simulink model "eVTOL_System"  (R2024b)
settings: Solver=FixedStepAuto  StartTime=0.0  StopTime=inf  RelTol=1e-3
undefined symbols (not defined in the file): airspeed, Battery, BCE12, BCE_Set_init, BMS_Controller_State, C, Cell10_P, Cell11_P, Cell12_P, Cell13_P, Cell14_P, Cell15_P, Cell16_P, Cell17_P, Cell18_P, Cell19_P, Cell1_N, Cell1_P, Cell20_P, Cell21_P, Cell22_P, Cell23_P, Cell24_P, Cell2_P, Cell3_P, Cell4_P, Cell5_P, Cell6_P, Cell7_P, Cell8_P, Cell9_P, Charging_State, CityMission, control, controlParams, ControlSampleTime, CriticalTiltAngle, currentFactor, CV_Gain, ddx, ddy, ddz, Device_01, Device_02, DiscIntNeverNeededParam, dx, dy, dz, Earth, env, F, F28379D_ADC_MaxCount, F28379D_ADC_Vmax, FixedWingMission, flightState, Foc_Ki_IxTcpu, Foc_Ki_S, Foc_Kp_I, Foc_Kp_S, fractalcoef ... (+68)
libraries: fl_lib x1115, nesl_utility x617, slrealtimeethercatlib x217, simulink x130, canmsglib x101, speedgoatlib_IO611_obsolete x91, slpidlib x49, mcbcontrolslib x44, slrealtimeutilitieslib x35, speedgoatlib_hdlCoder_IO3xx x31, dspstat3 x24, mcbpositiondecoderlib x12
(part 2 of 31)

== system eVTOL_System/Motor Drive/Controller3 ==
  Iab : Inport
  QAE_MIL_fbk : Inport  Port=2
  EnablePWM : Inport  Port=3
  Closed_Loop_FOC : Inport  Port=4
  Speed_CMD_RPM : Inport  Port=5
  Controller_Parameters : Inport  Port=6
  Controller_MIL : Subsystem  VariantControl=(default)
  Controller_fbk : Outport
  Simu_config : Outport  Port=2

== system eVTOL_System/Motor Drive/Controller_fbk_signals ==
  Controller_fbk : Inport
  Data Type Conversion : DataTypeConversion  OutDataTypeStr=boolean  SaturateOnIntegerOverflow=off  RndMeth=Floor
  Demux : Demux
  Terminator{,1..3} (4 alike) : Terminator
  wires:
  Demux/1 -> Terminator1/1  "Speed_fbk"
  Controller_fbk/1 -> Demux/1
  Demux/2 -> Terminator3/1  "Encoder_Pos_fbk"
  Demux/4 -> Data Type Conversion/1  "Spd_Pot_fdk"
  Demux/3 -> Terminator2/1  "Speed_Cmd_fbk"
  Data Type Conversion/1 -> Terminator/1  "Spd_pot_enable"

== system eVTOL_System/Motor Drive/Controller_fbk_signals1 ==
  Controller_fbk : Inport
  Data Type Conversion : DataTypeConversion  OutDataTypeStr=boolean  SaturateOnIntegerOverflow=off  RndMeth=Floor
  Demux : Demux
  Terminator{,1..3} (4 alike) : Terminator
  wires:
  Demux/1 -> Terminator1/1  "Speed_fbk"
  Controller_fbk/1 -> Demux/1
  Demux/2 -> Terminator3/1  "Encoder_Pos_fbk"
  Demux/4 -> Data Type Conversion/1  "Spd_Pot_fdk"
  Demux/3 -> Terminator2/1  "Speed_Cmd_fbk"
  Data Type Conversion/1 -> Terminator/1  "Spd_pot_enable"

== system eVTOL_System/Motor Drive/Controller_fbk_signals2 ==
  Controller_fbk : Inport
  Data Type Conversion : DataTypeConversion  OutDataTypeStr=boolean  SaturateOnIntegerOverflow=off  RndMeth=Floor
  Demux : Demux
  Terminator{,1..3} (4 alike) : Terminator
  wires:
  Demux/1 -> Terminator1/1  "Speed_fbk"
  Controller_fbk/1 -> Demux/1
  Demux/2 -> Terminator3/1  "Encoder_Pos_fbk"
  Demux/4 -> Data Type Conversion/1  "Spd_Pot_fdk"
  Demux/3 -> Terminator2/1  "Speed_Cmd_fbk"
  Data Type Conversion/1 -> Terminator/1  "Spd_pot_enable"

== system eVTOL_System/Motor Drive/Controller_fbk_signals3 ==
  Controller_fbk : Inport
  Data Type Conversion : DataTypeConversion  OutDataTypeStr=boolean  SaturateOnIntegerOverflow=off  RndMeth=Floor
  Demux : Demux
  Terminator{,1..3} (4 alike) : Terminator
  wires:
  Demux/1 -> Terminator1/1  "Speed_fbk"
  Controller_fbk/1 -> Demux/1
  Demux/2 -> Terminator3/1  "Encoder_Pos_fbk"
  Demux/4 -> Data Type Conversion/1  "Spd_Pot_fdk"
  Demux/3 -> Terminator2/1  "Speed_Cmd_fbk"
  Data Type Conversion/1 -> Terminator/1  "Spd_pot_enable"

== system eVTOL_System/Motor Drive/Fault Trigering ==
  AND : Logic  Inputs=3  IconShape=distinctive  AllPortsSameDT=off  OutDataTypeStr=boolean
  Bit to Integer Converter : simulink/Logic and Bit Operations/Bit to Integer Converter  nbits=32  bitOrder=LSB first  signedOutputValues=Unsigned  outDtype=uint32  outDtypeSigned=Inherit via internal rule
  Close_An : Constant  Value=0  OutDataTypeStr=boolean  SampleTime=Ts_UI
  Close_Ap : Constant  Value=0  OutDataTypeStr=boolean  SampleTime=Ts_UI
  Close_Bn : Constant  Value=0  OutDataTypeStr=boolean  SampleTime=Ts_UI
  Close_Bp : Constant  Value=0  OutDataTypeStr=boolean  SampleTime=Ts_UI
  Close_Cn : Constant  Value=0  OutDataTypeStr=boolean  SampleTime=Ts_UI
  Close_Cp : Constant  Value=0  OutDataTypeStr=boolean  SampleTime=Ts_UI
  Constant1 : Constant  Value=0  OutDataTypeStr=uint32
  Constant{14..15,20..25,32..36} (13 alike) : Constant  Value=0  OutDataTypeStr=boolean  SampleTime=Ts_UI
  Constant2 : Constant  OutDataTypeStr=boolean  SampleTime=Ts_UI
  Enable_Fault_UI : Constant  OutDataTypeStr=boolean  SampleTime=Ts_UI
  OR : Logic  Operator=OR  Inputs=18  IconShape=distinctive  AllPortsSameDT=off  OutDataTypeStr=boolean
  Open_An : Constant  Value=0  OutDataTypeStr=boolean  SampleTime=Ts_UI
  Open_Ap : Constant  Value=0  OutDataTypeStr=boolean  SampleTime=Ts_UI
  Open_Bn : Constant  Value=0  OutDataTypeStr=boolean  SampleTime=Ts_UI
  Open_Bp : Constant  Value=0  OutDataTypeStr=boolean  SampleTime=Ts_UI
  Open_Cn : Constant  Value=0  OutDataTypeStr=boolean  SampleTime=Ts_UI
  Open_Cp : Constant  Value=0  OutDataTypeStr=boolean  SampleTime=Ts_UI
  Short_A : Constant  Value=0  OutDataTypeStr=boolean  SampleTime=Ts_UI
  Short_AB : Constant  Value=0  OutDataTypeStr=boolean  SampleTime=Ts_UI
  Short_B : Constant  Value=0  OutDataTypeStr=boolean  SampleTime=Ts_UI
  Short_BC : Constant  Value=0  OutDataTypeStr=boolean  SampleTime=Ts_UI
  Short_C : Constant  Value=0  OutDataTypeStr=boolean  SampleTime=Ts_UI
  Short_CA : Constant  Value=0  OutDataTypeStr=boolean  SampleTime=Ts_UI
  Switch : Switch  Criteria=u2 > Threshold  SaturateOnIntegerOverflow=off  InputSameDT=off
  Terminator : Terminator
  Vector Concatenate : Concatenate  NumInputs=32
  Faults : Outport
  wires:
  Open_Cn/1 -> OR/12, Vector Concatenate/12
  Open_Cp/1 -> OR/9, Vector Concatenate/9
  Short_A/1 -> OR/1, Vector Concatenate/1
  Open_Bp/1 -> OR/8, Vector Concatenate/8
  Short_B/1 -> Vector Concatenate/2, OR/2
  Short_C/1 -> Vector Concatenate/3, OR/3
  Short_AB/1 -> Vector Concatenate/4, OR/4
  Short_BC/1 -> Vector Concatenate/5, OR/5
  Short_CA/1 -> OR/6, Vector Concatenate/6
  Constant36/1 -> Vector Concatenate/31
  Open_Bn/1 -> OR/11, Vector Concatenate/11
  Open_An/1 -> OR/10, Vector Concatenate/10
  Open_Ap/1 -> OR/7, Vector Concatenate/7
  Close_An/1 -> OR/16, Vector Concatenate/16
  Close_Ap/1 -> OR/13, Vector Concatenate/13
  Close_Cn/1 -> OR/18, Vector Concatenate/18
  Close_Bn/1 -> OR/17, Vector Concatenate/17
  Close_Cp/1 -> OR/15, Vector Concatenate/15
  Close_Bp/1 -> OR/14, Vector Concatenate/14
  Constant15/1 -> Vector Concatenate/24
  Constant14/1 -> Vector Concatenate/23
  Constant21/1 -> Vector Concatenate/20
  Constant20/1 -> Vector Concatenate/19
  Constant25/1 -> Vector Concatenate/26
  Constant24/1 -> Vector Concatenate/25
  Constant23/1 -> Vector Concatenate/22
  Constant22/1 -> Vector Concatenate/21
  Constant35/1 -> Vector Concatenate/30
  Constant34/1 -> Vector Concatenate/29
  Constant33/1 -> Vector Concatenate/28
  Constant32/1 -> Vector Concatenate/27
  Enable_Fault_UI/1 -> AND/3, Switch/2
  Vector Concatenate/1 -> Bit to Integer Converter/1
  Switch/1 -> Faults/1
  Bit to Integer Converter/1 -> Switch/1
  Constant1/1 -> Switch/3
  OR/1 -> AND/1
  AND/1 -> Terminator/1  "Fault_Present"
  Constant2/1 -> AND/2, Vector Concatenate/32

== system eVTOL_System/Motor Drive/Fault Trigering1 ==
  AND : Logic  Inputs=3  IconShape=distinctive  AllPortsSameDT=off  OutDataTypeStr=boolean
  Bit to Integer Converter : simulink/Logic and Bit Operations/Bit to Integer Converter  nbits=32  bitOrder=LSB first  signedOutputValues=Unsigned  outDtype=uint32  outDtypeSigned=Inherit via internal rule
  Close_An : Constant  Value=0  OutDataTypeStr=boolean  SampleTime=Ts_UI
  Close_Ap : Constant  Value=0  OutDataTypeStr=boolean  SampleTime=Ts_UI
  Close_Bn : Constant  Value=0  OutDataTypeStr=boolean  SampleTime=Ts_UI
  Close_Bp : Constant  Value=0  OutDataTypeStr=boolean  SampleTime=Ts_UI
  Close_Cn : Constant  Value=0  OutDataTypeStr=boolean  SampleTime=Ts_UI
  Close_Cp : Constant  Value=0  OutDataTypeStr=boolean  SampleTime=Ts_UI
  Constant1 : Constant  Value=0  OutDataTypeStr=uint32
  Constant{14..15,20..25,32..36} (13 alike) : Constant  Value=0  OutDataTypeStr=boolean  SampleTime=Ts_UI
  Constant2 : Constant  OutDataTypeStr=boolean  SampleTime=Ts_UI
  Enable_Fault_UI : Constant  OutDataTypeStr=boolean  SampleTime=Ts_UI
  OR : Logic  Operator=OR  Inputs=18  IconShape=distinctive  AllPortsSameDT=off  OutDataTypeStr=boolean
  Open_An : Constant  Value=0  OutDataTypeStr=boolean  SampleTime=Ts_UI
  Open_Ap : Constant  Value=0  OutDataTypeStr=boolean  SampleTime=Ts_UI
  Open_Bn : Constant  Value=0  OutDataTypeStr=boolean  SampleTime=Ts_UI
  Open_Bp : Constant  Value=0  OutDataTypeStr=boolean  SampleTime=Ts_UI
  Open_Cn : Constant  Value=0  OutDataTypeStr=boolean  SampleTime=Ts_UI
  Open_Cp : Constant  Value=0  OutDataTypeStr=boolean  SampleTime=Ts_UI
  Short_A : Constant  Value=0  OutDataTypeStr=boolean  SampleTime=Ts_UI
  Short_AB : Constant  Value=0  OutDataTypeStr=boolean  SampleTime=Ts_UI
  Short_B : Constant  Value=0  OutDataTypeStr=boolean  SampleTime=Ts_UI
  Short_BC : Constant  Value=0  OutDataTypeStr=boolean  SampleTime=Ts_UI
  Short_C : Constant  Value=0  OutDataTypeStr=boolean  SampleTime=Ts_UI
  Short_CA : Constant  Value=0  OutDataTypeStr=boolean  SampleTime=Ts_UI
  Switch : Switch  Criteria=u2 > Threshold  SaturateOnIntegerOverflow=off  InputSameDT=off
  Terminator : Terminator
  Vector Concatenate : Concatenate  NumInputs=32
  Faults : Outport
  wires:
  Open_Cn/1 -> OR/12, Vector Concatenate/12
  Open_Cp/1 -> OR/9, Vector Concatenate/9
  Short_A/1 -> OR/1, Vector Concatenate/1
  Open_Bp/1 -> OR/8, Vector Concatenate/8
  Short_B/1 -> Vector Concatenate/2, OR/2
  Short_C/1 -> Vector Concatenate/3, OR/3
  Short_AB/1 -> Vector Concatenate/4, OR/4
  Short_BC/1 -> Vector Concatenate/5, OR/5
  Short_CA/1 -> OR/6, Vector Concatenate/6
  Constant36/1 -> Vector Concatenate/31
  Open_Bn/1 -> OR/11, Vector Concatenate/11
  Open_An/1 -> OR/10, Vector Concatenate/10
  Open_Ap/1 -> OR/7, Vector Concatenate/7
  Close_An/1 -> OR/16, Vector Concatenate/16
  Close_Ap/1 -> OR/13, Vector Concatenate/13
  Close_Cn/1 -> OR/18, Vector Concatenate/18
  Close_Bn/1 -> OR/17, Vector Concatenate/17
  Close_Cp/1 -> OR/15, Vector Concatenate/15
  Close_Bp/1 -> OR/14, Vector Concatenate/14
  Constant15/1 -> Vector Concatenate/24
  Constant14/1 -> Vector Concatenate/23
  Constant21/1 -> Vector Concatenate/20
  Constant20/1 -> Vector Concatenate/19
  Constant25/1 -> Vector Concatenate/26
  Constant24/1 -> Vector Concatenate/25
  Constant23/1 -> Vector Concatenate/22
  Constant22/1 -> Vector Concatenate/21
  Constant35/1 -> Vector Concatenate/30
  Constant34/1 -> Vector Concatenate/29
  Constant33/1 -> Vector Concatenate/28
  Constant32/1 -> Vector Concatenate/27
  Enable_Fault_UI/1 -> AND/3, Switch/2
  Vector Concatenate/1 -> Bit to Integer Converter/1
  Switch/1 -> Faults/1
  Bit to Integer Converter/1 -> Switch/1
  Constant1/1 -> Switch/3
  OR/1 -> AND/1
  AND/1 -> Terminator/1  "Fault_Present"
  Constant2/1 -> AND/2, Vector Concatenate/32

== system eVTOL_System/Motor Drive/Fault Trigering2 ==
  AND : Logic  Inputs=3  IconShape=distinctive  AllPortsSameDT=off  OutDataTypeStr=boolean
  Bit to Integer Converter : simulink/Logic and Bit Operations/Bit to Integer Converter  nbits=32  bitOrder=LSB first  signedOutputValues=Unsigned  outDtype=uint32  outDtypeSigned=Inherit via internal rule
  Close_An : Constant  Value=0  OutDataTypeStr=boolean  SampleTime=Ts_UI
  Close_Ap : Constant  Value=0  OutDataTypeStr=boolean  SampleTime=Ts_UI
  Close_Bn : Constant  Value=0  OutDataTypeStr=boolean  SampleTime=Ts_UI
  Close_Bp : Constant  Value=0  OutDataTypeStr=boolean  SampleTime=Ts_UI
  Close_Cn : Constant  Value=0  OutDataTypeStr=boolean  SampleTime=Ts_UI
  Close_Cp : Constant  Value=0  OutDataTypeStr=boolean  SampleTime=Ts_UI
  Constant1 : Constant  Value=0  OutDataTypeStr=uint32
  Constant{14..15,20..25,32..36} (13 alike) : Constant  Value=0  OutDataTypeStr=boolean  SampleTime=Ts_UI
  Constant2 : Constant  OutDataTypeStr=boolean  SampleTime=Ts_UI
  Enable_Fault_UI : Constant  OutDataTypeStr=boolean  SampleTime=Ts_UI
  OR : Logic  Operator=OR  Inputs=18  IconShape=distinctive  AllPortsSameDT=off  OutDataTypeStr=boolean
  Open_An : Constant  Value=0  OutDataTypeStr=boolean  SampleTime=Ts_UI
  Open_Ap : Constant  Value=0  OutDataTypeStr=boolean  SampleTime=Ts_UI
  Open_Bn : Constant  Value=0  OutDataTypeStr=boolean  SampleTime=Ts_UI
  Open_Bp : Constant  Value=0  OutDataTypeStr=boolean  SampleTime=Ts_UI
  Open_Cn : Constant  Value=0  OutDataTypeStr=boolean  SampleTime=Ts_UI
  Open_Cp : Constant  Value=0  OutDataTypeStr=boolean  SampleTime=Ts_UI
  Short_A : Constant  Value=0  OutDataTypeStr=boolean  SampleTime=Ts_UI
  Short_AB : Constant  Value=0  OutDataTypeStr=boolean  SampleTime=Ts_UI
  Short_B : Constant  Value=0  OutDataTypeStr=boolean  SampleTime=Ts_UI
  Short_BC : Constant  Value=0  OutDataTypeStr=boolean  SampleTime=Ts_UI
  Short_C : Constant  Value=0  OutDataTypeStr=boolean  SampleTime=Ts_UI
  Short_CA : Constant  Value=0  OutDataTypeStr=boolean  SampleTime=Ts_UI
  Switch : Switch  Criteria=u2 > Threshold  SaturateOnIntegerOverflow=off  InputSameDT=off
  Terminator : Terminator
  Vector Concatenate : Concatenate  NumInputs=32
  Faults : Outport
  wires:
  Open_Cn/1 -> OR/12, Vector Concatenate/12
  Open_Cp/1 -> OR/9, Vector Concatenate/9
  Short_A/1 -> OR/1, Vector Concatenate/1
  Open_Bp/1 -> OR/8, Vector Concatenate/8
  Short_B/1 -> Vector Concatenate/2, OR/2
  Short_C/1 -> Vector Concatenate/3, OR/3
  Short_AB/1 -> Vector Concatenate/4, OR/4
  Short_BC/1 -> Vector Concatenate/5, OR/5
  Short_CA/1 -> OR/6, Vector Concatenate/6
  Constant36/1 -> Vector Concatenate/31
  Open_Bn/1 -> OR/11, Vector Concatenate/11
  Open_An/1 -> OR/10, Vector Concatenate/10
  Open_Ap/1 -> OR/7, Vector Concatenate/7
  Close_An/1 -> OR/16, Vector Concatenate/16
  Close_Ap/1 -> OR/13, Vector Concatenate/13
  Close_Cn/1 -> OR/18, Vector Concatenate/18
  Close_Bn/1 -> OR/17, Vector Concatenate/17
  Close_Cp/1 -> OR/15, Vector Concatenate/15
  Close_Bp/1 -> OR/14, Vector Concatenate/14
  Constant15/1 -> Vector Concatenate/24
  Constant14/1 -> Vector Concatenate/23
  Constant21/1 -> Vector Concatenate/20
  Constant20/1 -> Vector Concatenate/19
  Constant25/1 -> Vector Concatenate/26
  Constant24/1 -> Vector Concatenate/25
  Constant23/1 -> Vector Concatenate/22
  Constant22/1 -> Vector Concatenate/21
  Constant35/1 -> Vector Concatenate/30
  Constant34/1 -> Vector Concatenate/29
  Constant33/1 -> Vector Concatenate/28
  Constant32/1 -> Vector Concatenate/27
  Enable_Fault_UI/1 -> AND/3, Switch/2
  Vector Concatenate/1 -> Bit to Integer Converter/1
  Switch/1 -> Faults/1
  Bit to Integer Converter/1 -> Switch/1
  Constant1/1 -> Switch/3
  OR/1 -> AND/1
  AND/1 -> Terminator/1  "Fault_Present"
  Constant2/1 -> AND/2, Vector Concatenate/32

== system eVTOL_System/Motor Drive/Fault Trigering3 ==
  AND : Logic  Inputs=3  IconShape=distinctive  AllPortsSameDT=off  OutDataTypeStr=boolean
  Bit to Integer Converter : simulink/Logic and Bit Operations/Bit to Integer Converter  nbits=32  bitOrder=LSB first  signedOutputValues=Unsigned  outDtype=uint32  outDtypeSigned=Inherit via internal rule
  Close_An : Constant  Value=0  OutDataTypeStr=boolean  SampleTime=Ts_UI
  Close_Ap : Constant  Value=0  OutDataTypeStr=boolean  SampleTime=Ts_UI
  Close_Bn : Constant  Value=0  OutDataTypeStr=boolean  SampleTime=Ts_UI
  Close_Bp : Constant  Value=0  OutDataTypeStr=boolean  SampleTime=Ts_UI
  Close_Cn : Constant  Value=0  OutDataTypeStr=boolean  SampleTime=Ts_UI
  Close_Cp : Constant  Value=0  OutDataTypeStr=boolean  SampleTime=Ts_UI
  Constant1 : Constant  Value=0  OutDataTypeStr=uint32
  Constant{14..15,20..25,32..36} (13 alike) : Constant  Value=0  OutDataTypeStr=boolean  SampleTime=Ts_UI
  Constant2 : Constant  OutDataTypeStr=boolean  SampleTime=Ts_UI
  Enable_Fault_UI : Constant  OutDataTypeStr=boolean  SampleTime=Ts_UI
  OR : Logic  Operator=OR  Inputs=18  IconShape=distinctive  AllPortsSameDT=off  OutDataTypeStr=boolean
  Open_An : Constant  Value=0  OutDataTypeStr=boolean  SampleTime=Ts_UI
  Open_Ap : Constant  Value=0  OutDataTypeStr=boolean  SampleTime=Ts_UI
  Open_Bn : Constant  Value=0  OutDataTypeStr=boolean  SampleTime=Ts_UI
  Open_Bp : Constant  Value=0  OutDataTypeStr=boolean  SampleTime=Ts_UI
  Open_Cn : Constant  Value=0  OutDataTypeStr=boolean  SampleTime=Ts_UI
  Open_Cp : Constant  Value=0  OutDataTypeStr=boolean  SampleTime=Ts_UI
  Short_A : Constant  Value=0  OutDataTypeStr=boolean  SampleTime=Ts_UI
  Short_AB : Constant  Value=0  OutDataTypeStr=boolean  SampleTime=Ts_UI
  Short_B : Constant  Value=0  OutDataTypeStr=boolean  SampleTime=Ts_UI
  Short_BC : Constant  Value=0  OutDataTypeStr=boolean  SampleTime=Ts_UI
  Short_C : Constant  Value=0  OutDataTypeStr=boolean  SampleTime=Ts_UI
  Short_CA : Constant  Value=0  OutDataTypeStr=boolean  SampleTime=Ts_UI
  Switch : Switch  Criteria=u2 > Threshold  SaturateOnIntegerOverflow=off  InputSameDT=off
  Terminator : Terminator
  Vector Concatenate : Concatenate  NumInputs=32
  Faults : Outport
  wires:
  Open_Cn/1 -> OR/12, Vector Concatenate/12
  Open_Cp/1 -> OR/9, Vector Concatenate/9
  Short_A/1 -> OR/1, Vector Concatenate/1
  Open_Bp/1 -> OR/8, Vector Concatenate/8
  Short_B/1 -> Vector Concatenate/2, OR/2
  Short_C/1 -> Vector Concatenate/3, OR/3
  Short_AB/1 -> Vector Concatenate/4, OR/4
  Short_BC/1 -> Vector Concatenate/5, OR/5
  Short_CA/1 -> OR/6, Vector Concatenate/6
  Constant36/1 -> Vector Concatenate/31
  Open_Bn/1 -> OR/11, Vector Concatenate/11
  Open_An/1 -> OR/10, Vector Concatenate/10
  Open_Ap/1 -> OR/7, Vector Concatenate/7
  Close_An/1 -> OR/16, Vector Concatenate/16
  Close_Ap/1 -> OR/13, Vector Concatenate/13
  Close_Cn/1 -> OR/18, Vector Concatenate/18
  Close_Bn/1 -> OR/17, Vector Concatenate/17
  Close_Cp/1 -> OR/15, Vector Concatenate/15
  Close_Bp/1 -> OR/14, Vector Concatenate/14
  Constant15/1 -> Vector Concatenate/24
  Constant14/1 -> Vector Concatenate/23
  Constant21/1 -> Vector Concatenate/20
  Constant20/1 -> Vector Concatenate/19
  Constant25/1 -> Vector Concatenate/26
  Constant24/1 -> Vector Concatenate/25
  Constant23/1 -> Vector Concatenate/22
  Constant22/1 -> Vector Concatenate/21
  Constant35/1 -> Vector Concatenate/30
  Constant34/1 -> Vector Concatenate/29
  Constant33/1 -> Vector Concatenate/28
  Constant32/1 -> Vector Concatenate/27
  Enable_Fault_UI/1 -> AND/3, Switch/2
  Vector Concatenate/1 -> Bit to Integer Converter/1
  Switch/1 -> Faults/1
  Bit to Integer Converter/1 -> Switch/1
  Constant1/1 -> Switch/3
  OR/1 -> AND/1
  AND/1 -> Terminator/1  "Fault_Present"
  Constant2/1 -> AND/2, Vector Concatenate/32

== system eVTOL_System/Motor Drive/Motor Model Feedback ==
  Ia : Inport
  Ib : Inport  Port=2
  Ic : Inport  Port=3
  Motor_SPD_rads : Inport  Port=4
  Rate Transition{,1..3} (4 alike) : RateTransition  OutPortSampleTime=Ts_UI_fast
  Terminator{,1..3} (4 alike) : Terminator
  radsTOrpm : Gain  Gain=60/(2*pi)
  wires:
  Rate Transition1/1 -> Terminator/1  "Ia"
  Rate Transition3/1 -> Terminator2/1  "Ic"
  Rate Transition2/1 -> Terminator1/1  "Ib"
  Ib/1 -> Rate Transition2/1
  Ia/1 -> Rate Transition1/1
  Ic/1 -> Rate Transition3/1
  Motor_SPD_rads/1 -> Rate Transition/1
  radsTOrpm/1 -> Terminator3/1  "Motor Speed RPM"
  Rate Transition/1 -> radsTOrpm/1

== system eVTOL_System/Motor Drive/Motor Model Feedback1 ==
  Ia : Inport
  Ib : Inport  Port=2
  Ic : Inport  Port=3
  Motor_SPD_rads : Inport  Port=4
  Rate Transition{,1..3} (4 alike) : RateTransition  OutPortSampleTime=Ts_UI_fast
  Terminator{,1..3} (4 alike) : Terminator
  radsTOrpm : Gain  Gain=60/(2*pi)
  wires:
  Rate Transition1/1 -> Terminator/1  "Ia"
  Rate Transition3/1 -> Terminator2/1  "Ic"
  Rate Transition2/1 -> Terminator1/1  "Ib"
  Ib/1 -> Rate Transition2/1
  Ia/1 -> Rate Transition1/1
  Ic/1 -> Rate Transition3/1
  Motor_SPD_rads/1 -> Rate Transition/1
  radsTOrpm/1 -> Terminator3/1  "Motor Speed RPM"
  Rate Transition/1 -> radsTOrpm/1

== system eVTOL_System/Motor Drive/Motor Model Feedback2 ==
  Ia : Inport
  Ib : Inport  Port=2
  Ic : Inport  Port=3
  Motor_SPD_rads : Inport  Port=4
  Rate Transition{,1..3} (4 alike) : RateTransition  OutPortSampleTime=Ts_UI_fast
  Terminator{,1..3} (4 alike) : Terminator
  radsTOrpm : Gain  Gain=60/(2*pi)
  wires:
  Rate Transition1/1 -> Terminator/1  "Ia"
  Rate Transition3/1 -> Terminator2/1  "Ic"
  Rate Transition2/1 -> Terminator1/1  "Ib"
  Ib/1 -> Rate Transition2/1
  Ia/1 -> Rate Transition1/1
  Ic/1 -> Rate Transition3/1
  Motor_SPD_rads/1 -> Rate Transition/1
  radsTOrpm/1 -> Terminator3/1  "Motor Speed RPM"
  Rate Transition/1 -> radsTOrpm/1

== system eVTOL_System/Motor Drive/Motor Model Feedback3 ==
  Ia : Inport
  Ib : Inport  Port=2
  Ic : Inport  Port=3
  Motor_SPD_rads : Inport  Port=4
  Rate Transition{,1..3} (4 alike) : RateTransition  OutPortSampleTime=Ts_UI_fast
  Terminator{,1..3} (4 alike) : Terminator
  radsTOrpm : Gain  Gain=60/(2*pi)
  wires:
  Rate Transition1/1 -> Terminator/1  "Ia"
  Rate Transition3/1 -> Terminator2/1  "Ic"
  Rate Transition2/1 -> Terminator1/1  "Ib"
  Ib/1 -> Rate Transition2/1
  Ia/1 -> Rate Transition1/1
  Ic/1 -> Rate Transition3/1
  Motor_SPD_rads/1 -> Rate Transition/1
  radsTOrpm/1 -> Terminator3/1  "Motor Speed RPM"
  Rate Transition/1 -> radsTOrpm/1

== system eVTOL_System/Motor Drive/Three-Phase PMSM Drive ==
  V_dc : Inport
  Fault : Inport  Port=2
  LdTrq/Spd : Inport  Port=3
  Simu_config : Inport  Port=4
  PMSM and average inverter : Subsystem  VariantControl=str2num(get_param(['eVTOL_System/Motor Drive/SimulationVariant'], 'Value'))==1
  PMSM and inverter with switching dynamics : Subsystem  VariantControl=str2num(get_param(['eVTOL_System/Motor Drive/SimulationVariant'], 'Value'))>1
  Ia : Outport
  Ib : Outport  Port=2
  Ic : Outport  Port=3
  Motor_Spd : Outport  Port=4
  Motor_Angle : Outport  Port=5
  QAE_Pos_C : Outport  Port=6

== system eVTOL_System/Motor Drive/Three-Phase PMSM Drive1 ==
  V_dc : Inport
  Fault : Inport  Port=2
  LdTrq/Spd : Inport  Port=3
  Simu_config : Inport  Port=4
  PMSM and average inverter : Subsystem  VariantControl=(default)
  Ia : Outport
  Ib : Outport  Port=2
  Ic : Outport  Port=3
  Motor_Spd : Outport  Port=4
  Motor_Angle : Outport  Port=5
  QAE_Pos_C : Outport  Port=6

== system eVTOL_System/Motor Drive/Three-Phase PMSM Drive2 ==
  V_dc : Inport
  Fault : Inport  Port=2
  LdTrq/Spd : Inport  Port=3
  Simu_config : Inport  Port=4
  PMSM and average inverter : Subsystem  VariantControl=(default)
  Ia : Outport
  Ib : Outport  Port=2
  Ic : Outport  Port=3
  Motor_Spd : Outport  Port=4
  Motor_Angle : Outport  Port=5
  QAE_Pos_C : Outport  Port=6

== system eVTOL_System/Motor Drive/Three-Phase PMSM Drive3 ==
  V_dc : Inport
  Fault : Inport  Port=2
  LdTrq/Spd : Inport  Port=3
  Simu_config : Inport  Port=4
  PMSM and average inverter : Subsystem  VariantControl=(default)
  Ia : Outport
  Ib : Outport  Port=2
  Ic : Outport  Port=3
  Motor_Spd : Outport  Port=4
  Motor_Angle : Outport  Port=5
  QAE_Pos_C : Outport  Port=6

== system eVTOL_System/User Interface/ System User Interface ==
  note: Motor Currents [A]
  note: Motor Speed [RPM]
  note: Time [s]
  note: Battery Voltage [V]
  note: Battery Current [A]
  note: State of Charge of Battery Pack [%]
  note: Commanded Y (m)
  note: Commanded X (m)
  note: Hover Commands
  note: Commanded Altitude (m)
  note: Hover
  note: Transition
  note: Flight Mode
  note: Fixed Wing
  note: Back Transition
  note: Fixed Wing Commands
  note: Commanded Course
  note: Commanded Airspeed (m)
  note: Commanded Altitude
  note: Motor 1
  note: Motor 2
  note: Motor 3
  note: Motor 4
  note: Battery Power [kW]
  note: Manual Control
  note: System User Interface
  Circular Gauge1 : CustomWebBlock  LabelPosition=Hide  ShowInitialText=on  Configuration="{\"components\":[{\"name\":\"CircularScaleComponent\",\"settings\":{\"bounds\":{\"max\":450,\"min\":95,\"tickInterval\":\"auto\"},\"direction\":\"cw\",\"flipLimits\":0,\"innerRadius\":0.75,\"internalTickHeightScaleFactor\":1,\"labelColor\":[204,204,204],\"labelFont\":{\"font\":\"Arial\",\"fontSize\":12},\"labelRadius\":0.528,\"labelTransparency\":1,\"minorTickHeightScaleFactor\":0.2,\"needleImage\":{\"size\":[0,0],\"src\":\"\"},\"needleOffset\":[0,0],\"needleOrientation\":-45,\"needleRotation\":0,\"needleSize\":{\"height\":0,\"width\":0},\"outerRadius\":0.9,\"position\":[0.06487573099415204,0.0561242816091954,0.8917923850574713,0.8786549707602339],\"referencePoint\":\"auto\",\"scaleAngle\":270,\"scaleAngleOffset\":135,\"scaleColors\":[],\"scaleColorsSize\":0.2,\"scaleDirection\":\"CW\",\"scalePosition\":[0,0,1,1],\"showLabels\":1,\"showMinorTicks\":1,\"showSpanLine\":true,\"showTicks\":false,\"tickColor\":[0,114,189],\"tickTransparency\":1,\"valueBarColor\":[0,114,189],\"valueBarPosition\":[0,0,1,1],\"valueBarSize\":0.2,\"valueBarTransparency\":1}},{\"name\":\"BackgroundImageComponent\",\"settings\":{\"image\":{\"size\":[0,0],\"src\":\"default\"},\"position\":[0,0,1,1],\"scaleMode\":\"0\"}},{\"name\":\"ForegroundImageComponent\",\"settings\":{\"image\":{\"size\":[0,0],\"src\":\"default\",\"srcOrientation\":[]},\"isForeground\":1,\"position\":[0,0,1,1],\"scaleMode\":\"0\"}}],\"settings\":{\"BindingType\":\"signal\",\"aspectRatio\":1.032258064516129,\"backgroundColor\":[0,0,0,\"1\"],\"backgroundOffset\":0.14,\"backgroundOpacity\":1,\"direction\":\"cw\",\"fixedAspectRatio\":\"on\",\"flipLimits\":0,\"orientation\":\"horizontal\",\"showBackgroundColor\":false,\"value\":0,\"version\":\"R2022b\"},\"type\":\"CircularGauge\"}"  CustomBackgroundColor="{\"color\":[0.1568627450980392,0.1607843137254902,0.20784313725490197],\"show\":true}"
  Circular Gauge3 : CustomWebBlock  LabelPosition=Hide  ShowInitialText=on  Configuration="{\"components\":[{\"name\":\"CircularScaleComponent\",\"settings\":{\"bounds\":{\"max\":450,\"min\":95,\"tickInterval\":\"auto\"},\"direction\":\"cw\",\"flipLimits\":0,\"innerRadius\":0.75,\"internalTickHeightScaleFactor\":1,\"labelColor\":[204,204,204],\"labelFont\":{\"font\":\"Arial\",\"fontSize\":12},\"labelRadius\":0.528,\"labelTransparency\":1,\"minorTickHeightScaleFactor\":0.2,\"needleImage\":{\"size\":[0,0],\"src\":\"\"},\"needleOffset\":[0,0],\"needleOrientation\":-45,\"needleRotation\":0,\"needleSize\":{\"height\":0,\"width\":0},\"outerRadius\":0.9,\"position\":[0.06487573099415204,0.0561242816091954,0.8917923850574713,0.8786549707602339],\"referencePoint\":\"auto\",\"scaleAngle\":270,\"scaleAngleOffset\":135,\"scaleColors\":[],\"scaleColorsSize\":0.2,\"scaleDirection\":\"CW\",\"scalePosition\":[0,0,1,1],\"showLabels\":1,\"showMinorTicks\":1,\"showSpanLine\":true,\"showTicks\":false,\"tickColor\":[0,114,189],\"tickTransparency\":1,\"valueBarColor\":[0,114,189],\"valueBarPosition\":[0,0,1,1],\"valueBarSize\":0.2,\"valueBarTransparency\":1}},{\"name\":\"BackgroundImageComponent\",\"settings\":{\"image\":{\"size\":[0,0],\"src\":\"default\"},\"position\":[0,0,1,1],\"scaleMode\":\"0\"}},{\"name\":\"ForegroundImageComponent\",\"settings\":{\"image\":{\"size\":[0,0],\"src\":\"default\",\"srcOrientation\":[]},\"isForeground\":1,\"position\":[0,0,1,1],\"scaleMode\":\"0\"}}],\"settings\":{\"BindingType\":\"signal\",\"aspectRatio\":1.032258064516129,\"backgroundColor\":[0,0,0,\"1\"],\"backgroundOffset\":0.14,\"backgroundOpacity\":1,\"direction\":\"cw\",\"fixedAspectRatio\":\"on\",\"flipLimits\":0,\"orientation\":\"horizontal\",\"showBackgroundColor\":false,\"value\":0,\"version\":\"R2022b\"},\"type\":\"CircularGauge\"}"  CustomBackgroundColor="{\"color\":[0.1568627450980392,0.1607843137254902,0.20784313725490197],\"show\":true}"
  Dashboard Scope1 : DashboardScope  ShowInitialText=off  TimeSpan=0.10000000000000001  Ymin=-50  Ymax=50  ScaleAtStop=off  UpdateMode=Scroll
  Gauge{1..4} (4 alike) : CircularGaugeBlock  LabelPosition=Hide  ScaleMin=-1500  ScaleMax=1500
  Lamp : LampBlock  LabelPosition=Hide
  Pack_Voltage : DisplayBlock  LabelPosition=Hide  Format=Integer  Transparency=1  Opacity=0
  Pack_Voltage1 : DisplayBlock  LabelPosition=Hide  Format=Integer  Transparency=1  Opacity=0
  SOC : DisplayBlock  LabelPosition=Hide  Format=Integer  Transparency=1  Opacity=0  FormatString=%1.1f
  SOC1 : DisplayBlock  LabelPosition=Hide  Format=Integer  Transparency=1  Opacity=0  FormatString=%1.1f
  Slider1 : SliderBlock  LabelPosition=Hide  ScaleMax=50  TickInterval=5
  Slider2 : SliderBlock  LabelPosition=Hide  ScaleMin=-30  ScaleMax=30  TickInterval=5
  Slider3 : SliderBlock  LabelPosition=Hide  ScaleMin=-30  ScaleMax=30  TickInterval=5
  Slider4 : SliderBlock  LabelPosition=Hide  ScaleMax=3  TickInterval=1
  Slider5 : SliderBlock  LabelPosition=Hide  ScaleMin=-30  ScaleMax=30  TickInterval=5
  Slider6 : SliderBlock  LabelPosition=Hide  ScaleMin=-100  TickInterval=10
  Slider7 : SliderBlock  LabelPosition=Hide  ScaleMin=10  ScaleMax=30  TickInterval=5
  wdwqdwqdwq : CustomWebBlock  LabelPosition=Hide  ShowInitialText=on  Configuration="{\"components\":[{\"name\":\"CircularScaleComponent\",\"settings\":{\"bounds\":{\"max\":100,\"min\":0,\"tickInterval\":\"auto\"},\"direction\":\"cw\",\"flipLimits\":0,\"innerRadius\":0.75,\"internalTickHeightScaleFactor\":1,\"labelColor\":[204,204,204],\"labelFont\":{\"font\":\"Arial\",\"fontSize\":12},\"labelRadius\":0.528,\"labelTransparency\":1,\"minorTickHeightScaleFactor\":0.2,\"needleImage\":{\"size\":[0,0],\"src\":\"\"},\"needleOffset\":[0,0],\"needleOrientation\":-45,\"needleRotation\":0,\"needleSize\":{\"height\":0,\"width\":0},\"outerRadius\":0.9,\"position\":[0.06487573099415204,0.0561242816091954,0.8917923850574713,0.8786549707602339],\"referencePoint\":\"auto\",\"scaleAngle\":270,\"scaleAngleOffset\":135,\"scaleColors\":[],\"scaleColorsSize\":0.2,\"scaleDirection\":\"CW\",\"scalePosition\":[0,0,1,1],\"showLabels\":1,\"showMinorTicks\":1,\"showSpanLine\":true,\"showTicks\":false,\"tickColor\":[0,114,189],\"tickTransparency\":1,\"valueBarColor\":[0,114,189],\"valueBarPosition\":[0,0,1,1],\"valueBarSize\":0.2,\"valueBarTransparency\":1}},{\"name\":\"BackgroundImageComponent\",\"settings\":{\"image\":{\"size\":[0,0],\"src\":\"default\"},\"position\":[0,0,1,1],\"scaleMode\":\"0\"}},{\"name\":\"ForegroundImageComponent\",\"settings\":{\"image\":{\"size\":[0,0],\"src\":\"default\",\"srcOrientation\":[]},\"isForeground\":1,\"position\":[0,0,1,1],\"scaleMode\":\"0\"}}],\"settings\":{\"BindingType\":\"signal\",\"aspectRatio\":1.032258064516129,\"backgroundColor\":[0,0,0,\"1\"],\"backgroundOffset\":0.14,\"backgroundOpacity\":1,\"direction\":\"cw\",\"fixedAspectRatio\":\"on\",\"flipLimits\":0,\"orientation\":\"horizontal\",\"showBackgroundColor\":false,\"value\":0,\"version\":\"R2022b\"},\"type\":\"CircularGauge\"}"  CustomBackgroundColor="{\"color\":[0.1568627450980392,0.1607843137254902,0.20784313725490197],\"show\":true}"
  wdwqdwqdwq1 : CustomWebBlock  LabelPosition=Hide  ShowInitialText=on  Configuration="{\"components\":[{\"name\":\"CircularScaleComponent\",\"settings\":{\"bounds\":{\"max\":200,\"min\":0,\"tickInterval\":\"auto\"},\"direction\":\"cw\",\"flipLimits\":0,\"innerRadius\":0.75,\"internalTickHeightScaleFactor\":1,\"labelColor\":[204,204,204],\"labelFont\":{\"font\":\"Arial\",\"fontSize\":12},\"labelRadius\":0.528,\"labelTransparency\":1,\"minorTickHeightScaleFactor\":0.2,\"needleImage\":{\"size\":[0,0],\"src\":\"\"},\"needleOffset\":[0,0],\"needleOrientation\":-45,\"needleRotation\":0,\"needleSize\":{\"height\":0,\"width\":0},\"outerRadius\":0.9,\"position\":[0.06487573099415204,0.0561242816091954,0.8917923850574713,0.8786549707602339],\"referencePoint\":\"auto\",\"scaleAngle\":270,\"scaleAngleOffset\":135,\"scaleColors\":[],\"scaleColorsSize\":0.2,\"scaleDirection\":\"CW\",\"scalePosition\":[0,0,1,1],\"showLabels\":1,\"showMinorTicks\":1,\"showSpanLine\":true,\"showTicks\":false,\"tickColor\":[0,114,189],\"tickTransparency\":1,\"valueBarColor\":[0,114,189],\"valueBarPosition\":[0,0,1,1],\"valueBarSize\":0.2,\"valueBarTransparency\":1}},{\"name\":\"BackgroundImageComponent\",\"settings\":{\"image\":{\"size\":[0,0],\"src\":\"default\"},\"position\":[0,0,1,1],\"scaleMode\":\"0\"}},{\"name\":\"ForegroundImageComponent\",\"settings\":{\"image\":{\"size\":[0,0],\"src\":\"default\",\"srcOrientation\":[]},\"isForeground\":1,\"position\":[0,0,1,1],\"scaleMode\":\"0\"}}],\"settings\":{\"BindingType\":\"signal\",\"aspectRatio\":1.032258064516129,\"backgroundColor\":[0,0,0,\"1\"],\"backgroundOffset\":0.14,\"backgroundOpacity\":1,\"direction\":\"cw\",\"fixedAspectRatio\":\"on\",\"flipLimits\":0,\"orientation\":\"horizontal\",\"showBackgroundColor\":false,\"value\":0,\"version\":\"R2022b\"},\"type\":\"CircularGauge\"}"  CustomBackgroundColor="{\"color\":[0.1568627450980392,0.1607843137254902,0.20784313725490197],\"show\":true}"
